simulink model "airspeed_throttle"  (R2017a)
settings: Solver=VariableStepAuto  StartTime=0.0  StopTime=10.0  RelTol=1e-3
values from neighbouring files (symbols this model uses):
  a_V1 = P.rho*Va*P.S_wing/P.mass*(P.C_D_0 + P.C_D_alpha*alpha +      P.C_D_delta_e*delta_e) + P.rho*P.S_wing*P.C_prop*Va/P.mass    [computeRollGains.m]    (also in compute_gains.m = P.rho*Va*P.S_wing/P.mass*(P.C_D_0 + P.C_D_alpha*alpha_trim +)
  a_V2 = P.rho*P.S_prop*P.C_prop*P.k_motor^2*delta_t/P.mass    [computeRollGains.m]    (also in compute_gains.m = P.rho*P.S_prop*P.C_prop*P.k_motor^2*delta_t_trim/P.mass)
undefined symbols (not defined in the file or in its folder): ki_V, kp_V
settings Model: Creator=pizzaslayer  LastModifiedBy=pizzaslayer

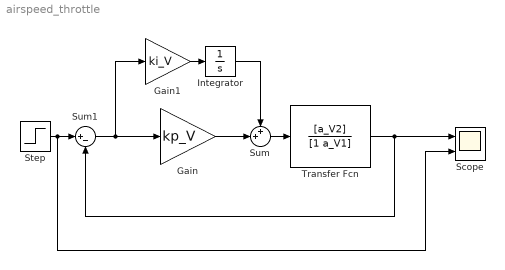
== system airspeed_throttle ==
  Gain : Gain  Gain=kp_V
  Gain1 : Gain  Gain=ki_V
  Integrator : Integrator
  Scope : Scope  NumInputPorts=2
  Step : Step  SampleTime=0
  Sum : Sum  Inputs=++|
  Sum1 : Sum  Inputs=|+-
  Transfer Fcn : TransferFcn  Numerator=[a_V2]  Denominator=[1 a_V1]
  wires:
  Gain1/1 -> Integrator/1
  Step/1 -> Scope/2, Sum1/1
  Sum1/1 -> Gain1/1, Gain/1
  Integrator/1 -> Sum/1
  Gain/1 -> Sum/2
  Transfer Fcn/1 -> Scope/1, Sum1/2
  Sum/1 -> Transfer Fcn/1
